simulink model "ICRA_demo_ver2"  (R2016a)
settings: Solver=FixedStepDiscrete  StartTime=0.0  StopTime=Inf  FixedStep=Ts  RelTol=1e-3
InitFcn:
  | Ts = 1/4000;
  | Ts2 = 1/1000;
  | Tmpc = 1/40;
  | 
  | q_off = calib.q_off;
  | q_init = calib.q_init;
libraries: xpcethercatlib x109, slrtlib x18
(part 2 of 2)

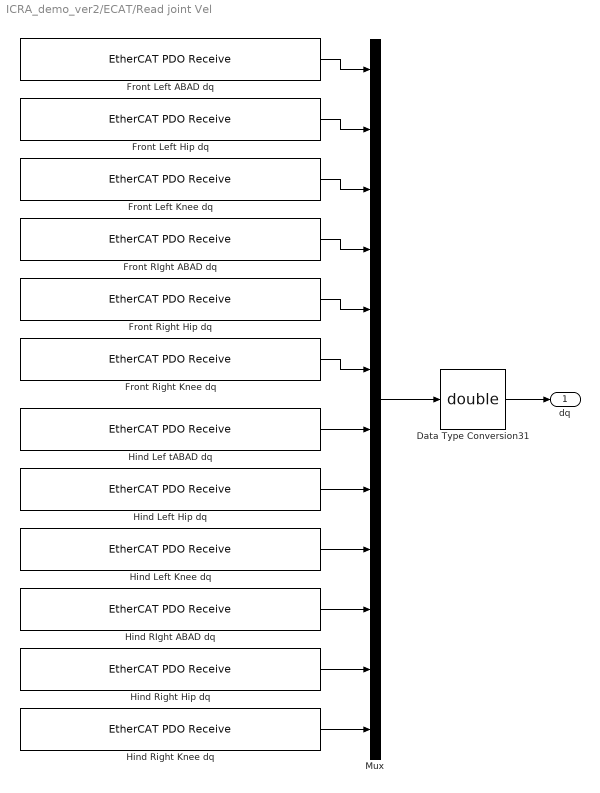
== system ICRA_demo_ver2/ECAT/Read joint Vel ==
  Data Type Conversion31 : DataTypeConversion  OutDataTypeStr=double
  Front Left ABAD dq : xpcethercatlib/EtherCAT PDO Receive  Priority=2  sig_name=Drive 1 (Elmo Drive).Inputs.Velocity actual value  sig_offset=920  sig_type=int32  type_size=32  sig_dim=1  device_id=0  sample_time=0.000250
  Front Left Hip dq : xpcethercatlib/EtherCAT PDO Receive  Priority=2  sig_name=Drive 2 (Elmo Drive).Inputs.Velocity actual value  sig_offset=1048  sig_type=int32  type_size=32  sig_dim=1  device_id=0  sample_time=0.000250
  Front Left Knee dq : xpcethercatlib/EtherCAT PDO Receive  Priority=2  sig_name=Drive 3 (Elmo Drive).Inputs.Velocity actual value  sig_offset=1176  sig_type=int32  type_size=32  sig_dim=1  device_id=0  sample_time=0.000250
  Front RIght ABAD dq : xpcethercatlib/EtherCAT PDO Receive  Priority=2  sig_name=Drive 13 (Elmo Drive).Inputs.Velocity actual value  sig_offset=2328  sig_type=int32  type_size=32  sig_dim=1  device_id=0  sample_time=0.000250
  Front Right Hip dq : xpcethercatlib/EtherCAT PDO Receive  Priority=2  sig_name=Drive 5 (Elmo Drive).Inputs.Velocity actual value  sig_offset=1304  sig_type=int32  type_size=32  sig_dim=1  device_id=0  sample_time=0.000250
  Front Right Knee dq : xpcethercatlib/EtherCAT PDO Receive  Priority=2  sig_name=Drive 6 (Elmo Drive).Inputs.Velocity actual value  sig_offset=1432  sig_type=int32  type_size=32  sig_dim=1  device_id=0  sample_time=0.000250
  Hind Lef tABAD dq : xpcethercatlib/EtherCAT PDO Receive  Priority=2  sig_name=Drive 7 (Elmo Drive).Inputs.Velocity actual value  sig_offset=1560  sig_type=int32  type_size=32  sig_dim=1  device_id=0  sample_time=0.000250
  Hind Left Hip dq : xpcethercatlib/EtherCAT PDO Receive  Priority=2  sig_name=Drive 8 (Elmo Drive).Inputs.Velocity actual value  sig_offset=1688  sig_type=int32  type_size=32  sig_dim=1  device_id=0  sample_time=0.000250
  Hind Left Knee dq : xpcethercatlib/EtherCAT PDO Receive  Priority=2  sig_name=Drive 9 (Elmo Drive).Inputs.Velocity actual value  sig_offset=1816  sig_type=int32  type_size=32  sig_dim=1  device_id=0  sample_time=0.000250
  Hind RIght ABAD dq : xpcethercatlib/EtherCAT PDO Receive  Priority=2  sig_name=Drive 10 (Elmo Drive).Inputs.Velocity actual value  sig_offset=1944  sig_type=int32  type_size=32  sig_dim=1  device_id=0  sample_time=0.000250
  Hind Right Hip dq : xpcethercatlib/EtherCAT PDO Receive  Priority=2  sig_name=Drive 11 (Elmo Drive).Inputs.Velocity actual value  sig_offset=2072  sig_type=int32  type_size=32  sig_dim=1  device_id=0  sample_time=0.000250
  Hind Right Knee dq : xpcethercatlib/EtherCAT PDO Receive  Priority=2  sig_name=Drive 12 (Elmo Drive).Inputs.Velocity actual value  sig_offset=2200  sig_type=int32  type_size=32  sig_dim=1  device_id=0  sample_time=0.000250
  Mux : Mux  Inputs=12
  dq : Outport
  wires:
  Hind Right Knee dq/1 -> Mux/12
  Hind Right Hip dq/1 -> Mux/11
  Hind RIght ABAD dq/1 -> Mux/10
  Hind Left Knee dq/1 -> Mux/9
  Hind Left Hip dq/1 -> Mux/8
  Hind Lef tABAD dq/1 -> Mux/7
  Front Right Knee dq/1 -> Mux/6
  Front Left Hip dq/1 -> Mux/2
  Front Left Knee dq/1 -> Mux/3
  Front RIght ABAD dq/1 -> Mux/4
  Front Right Hip dq/1 -> Mux/5
  Mux/1 -> Data Type Conversion31/1
  Data Type Conversion31/1 -> dq/1
  Front Left ABAD dq/1 -> Mux/1

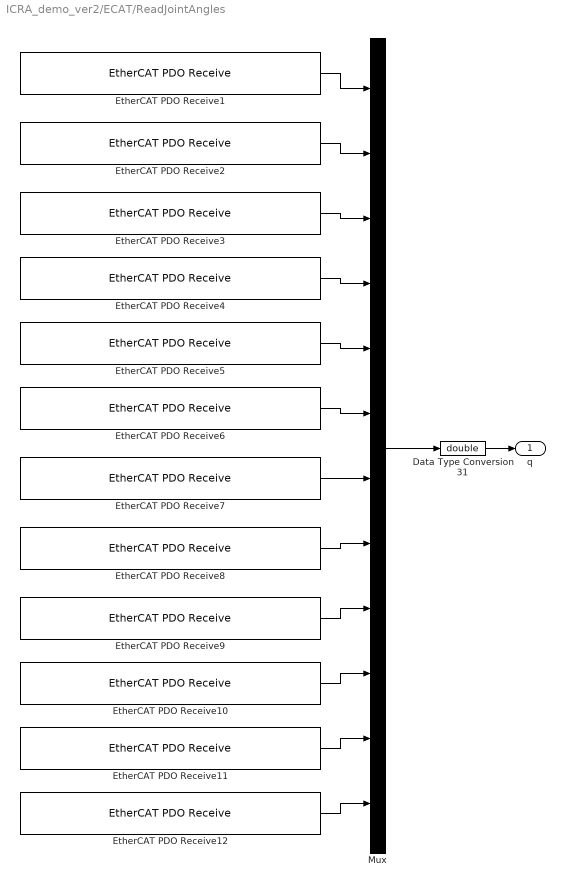
== system ICRA_demo_ver2/ECAT/ReadJointAngles ==
  Data Type Conversion31 : DataTypeConversion  OutDataTypeStr=double
  EtherCAT PDO Receive1 : xpcethercatlib/EtherCAT PDO Receive  Priority=2  sig_name=Drive 1 (Elmo Drive).Inputs.Position actual value  sig_offset=856  sig_type=int32  type_size=32  sig_dim=1  device_id=0  sample_time=0.000250
  EtherCAT PDO Receive10 : xpcethercatlib/EtherCAT PDO Receive  Priority=2  sig_name=Drive 10 (Elmo Drive).Inputs.Position actual value  sig_offset=1880  sig_type=int32  type_size=32  sig_dim=1  device_id=0  sample_time=0.000250
  EtherCAT PDO Receive11 : xpcethercatlib/EtherCAT PDO Receive  Priority=2  sig_name=Drive 11 (Elmo Drive).Inputs.Position actual value  sig_offset=2008  sig_type=int32  type_size=32  sig_dim=1  device_id=0  sample_time=0.000250
  EtherCAT PDO Receive12 : xpcethercatlib/EtherCAT PDO Receive  Priority=2  sig_name=Drive 12 (Elmo Drive).Inputs.Position actual value  sig_offset=2136  sig_type=int32  type_size=32  sig_dim=1  device_id=0  sample_time=0.000250
  EtherCAT PDO Receive2 : xpcethercatlib/EtherCAT PDO Receive  Priority=2  sig_name=Drive 2 (Elmo Drive).Inputs.Position actual value  sig_offset=984  sig_type=int32  type_size=32  sig_dim=1  device_id=0  sample_time=0.000250
  EtherCAT PDO Receive3 : xpcethercatlib/EtherCAT PDO Receive  Priority=2  sig_name=Drive 3 (Elmo Drive).Inputs.Position actual value  sig_offset=1112  sig_type=int32  type_size=32  sig_dim=1  device_id=0  sample_time=0.000250
  EtherCAT PDO Receive4 : xpcethercatlib/EtherCAT PDO Receive  Priority=2  sig_name=Drive 13 (Elmo Drive).Inputs.Position actual value  sig_offset=2264  sig_type=int32  type_size=32  sig_dim=1  device_id=0  sample_time=0.000250
  EtherCAT PDO Receive5 : xpcethercatlib/EtherCAT PDO Receive  Priority=2  sig_name=Drive 5 (Elmo Drive).Inputs.Position actual value  sig_offset=1240  sig_type=int32  type_size=32  sig_dim=1  device_id=0  sample_time=0.000250
  EtherCAT PDO Receive6 : xpcethercatlib/EtherCAT PDO Receive  Priority=2  sig_name=Drive 6 (Elmo Drive).Inputs.Position actual value  sig_offset=1368  sig_type=int32  type_size=32  sig_dim=1  device_id=0  sample_time=0.000250
  EtherCAT PDO Receive7 : xpcethercatlib/EtherCAT PDO Receive  Priority=2  sig_name=Drive 7 (Elmo Drive).Inputs.Position actual value  sig_offset=1496  sig_type=int32  type_size=32  sig_dim=1  device_id=0  sample_time=0.000250
  EtherCAT PDO Receive8 : xpcethercatlib/EtherCAT PDO Receive  Priority=2  sig_name=Drive 8 (Elmo Drive).Inputs.Position actual value  sig_offset=1624  sig_type=int32  type_size=32  sig_dim=1  device_id=0  sample_time=0.000250
  EtherCAT PDO Receive9 : xpcethercatlib/EtherCAT PDO Receive  Priority=2  sig_name=Drive 9 (Elmo Drive).Inputs.Position actual value  sig_offset=1752  sig_type=int32  type_size=32  sig_dim=1  device_id=0  sample_time=0.000250
  Mux : Mux  Inputs=12
  q : Outport
  wires:
  EtherCAT PDO Receive12/1 -> Mux/12
  EtherCAT PDO Receive11/1 -> Mux/11
  EtherCAT PDO Receive10/1 -> Mux/10
  EtherCAT PDO Receive9/1 -> Mux/9
  EtherCAT PDO Receive8/1 -> Mux/8
  EtherCAT PDO Receive7/1 -> Mux/7
  EtherCAT PDO Receive6/1 -> Mux/6
  EtherCAT PDO Receive1/1 -> Mux/1
  EtherCAT PDO Receive2/1 -> Mux/2
  EtherCAT PDO Receive3/1 -> Mux/3
  EtherCAT PDO Receive4/1 -> Mux/4
  EtherCAT PDO Receive5/1 -> Mux/5
  Mux/1 -> Data Type Conversion31/1
  Data Type Conversion31/1 -> q/1

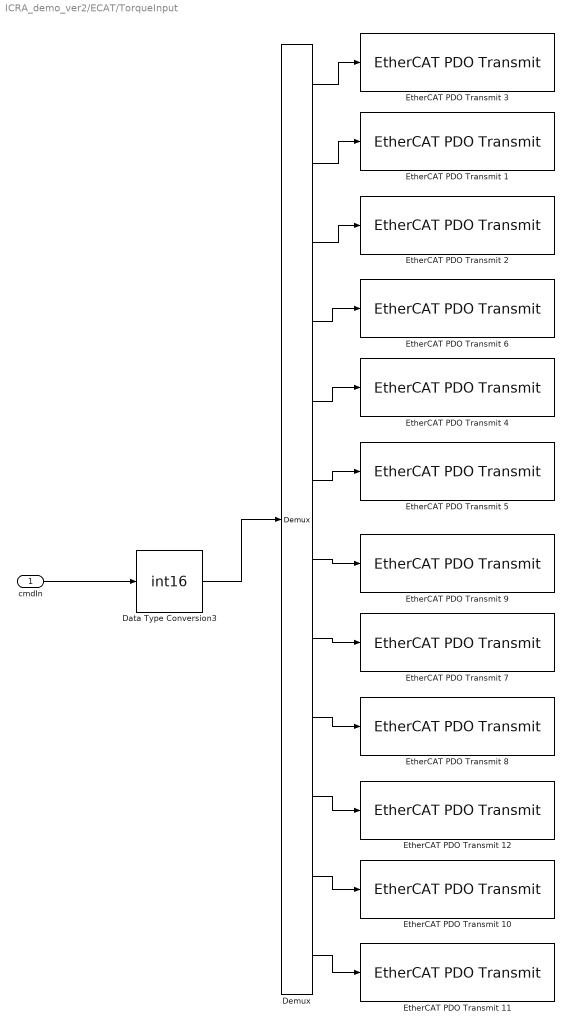
== system ICRA_demo_ver2/ECAT/TorqueInput ==
  cmdIn : Inport
  Data Type Conversion3 : DataTypeConversion  OutDataTypeStr=int16
  Demux : Demux  Outputs=12
  EtherCAT PDO Transmit 1 : xpcethercatlib/EtherCAT PDO Transmit   Priority=3  sig_name=Drive 2 (Elmo Drive).Outputs.Target Torque  sig_offset=1048  sig_type=int16  type_size=16  sig_dim=1  device_id=0  sample_time=0.000250
  EtherCAT PDO Transmit 10 : xpcethercatlib/EtherCAT PDO Transmit   Priority=3  sig_name=Drive 11 (Elmo Drive).Outputs.Target Torque  sig_offset=2072  sig_type=int16  type_size=16  sig_dim=1  device_id=0  sample_time=0.000250
  EtherCAT PDO Transmit 11 : xpcethercatlib/EtherCAT PDO Transmit   Priority=3  sig_name=Drive 12 (Elmo Drive).Outputs.Target Torque  sig_offset=2200  sig_type=int16  type_size=16  sig_dim=1  device_id=0  sample_time=0.000250
  EtherCAT PDO Transmit 12 : xpcethercatlib/EtherCAT PDO Transmit   Priority=3  sig_name=Drive 10 (Elmo Drive).Outputs.Target Torque  sig_offset=1944  sig_type=int16  type_size=16  sig_dim=1  device_id=0  sample_time=0.000250
  EtherCAT PDO Transmit 2 : xpcethercatlib/EtherCAT PDO Transmit   Priority=3  sig_name=Drive 3 (Elmo Drive).Outputs.Target Torque  sig_offset=1176  sig_type=int16  type_size=16  sig_dim=1  device_id=0  sample_time=0.000250
  EtherCAT PDO Transmit 3 : xpcethercatlib/EtherCAT PDO Transmit   Priority=3  sig_name=Drive 1 (Elmo Drive).Outputs.Target Torque  sig_offset=920  sig_type=int16  type_size=16  sig_dim=1  device_id=0  sample_time=0.000250
  EtherCAT PDO Transmit 4 : xpcethercatlib/EtherCAT PDO Transmit   Priority=3  sig_name=Drive 5 (Elmo Drive).Outputs.Target Torque  sig_offset=1304  sig_type=int16  type_size=16  sig_dim=1  device_id=0  sample_time=0.000250
  EtherCAT PDO Transmit 5 : xpcethercatlib/EtherCAT PDO Transmit   Priority=3  sig_name=Drive 6 (Elmo Drive).Outputs.Target Torque  sig_offset=1432  sig_type=int16  type_size=16  sig_dim=1  device_id=0  sample_time=0.000250
  EtherCAT PDO Transmit 6 : xpcethercatlib/EtherCAT PDO Transmit   Priority=3  sig_name=Drive 13 (Elmo Drive).Outputs.Target Torque  sig_offset=2328  sig_type=int16  type_size=16  sig_dim=1  device_id=0  sample_time=0.000250
  EtherCAT PDO Transmit 7 : xpcethercatlib/EtherCAT PDO Transmit   Priority=3  sig_name=Drive 8 (Elmo Drive).Outputs.Target Torque  sig_offset=1688  sig_type=int16  type_size=16  sig_dim=1  device_id=0  sample_time=0.000250
  EtherCAT PDO Transmit 8 : xpcethercatlib/EtherCAT PDO Transmit   Priority=3  sig_name=Drive 9 (Elmo Drive).Outputs.Target Torque  sig_offset=1816  sig_type=int16  type_size=16  sig_dim=1  device_id=0  sample_time=0.000250
  EtherCAT PDO Transmit 9 : xpcethercatlib/EtherCAT PDO Transmit   Priority=3  sig_name=Drive 7 (Elmo Drive).Outputs.Target Torque  sig_offset=1560  sig_type=int16  type_size=16  sig_dim=1  device_id=0  sample_time=0.000250
  wires:
  Demux/3 -> EtherCAT PDO Transmit 2/1
  Demux/2 -> EtherCAT PDO Transmit 1/1
  Demux/1 -> EtherCAT PDO Transmit 3/1
  cmdIn/1 -> Data Type Conversion3/1
  Data Type Conversion3/1 -> Demux/1
  Demux/4 -> EtherCAT PDO Transmit 6/1
  Demux/5 -> EtherCAT PDO Transmit 4/1
  Demux/6 -> EtherCAT PDO Transmit 5/1
  Demux/7 -> EtherCAT PDO Transmit 9/1
  Demux/8 -> EtherCAT PDO Transmit 7/1
  Demux/9 -> EtherCAT PDO Transmit 8/1
  Demux/10 -> EtherCAT PDO Transmit 12/1
  Demux/11 -> EtherCAT PDO Transmit 10/1
  Demux/12 -> EtherCAT PDO Transmit 11/1

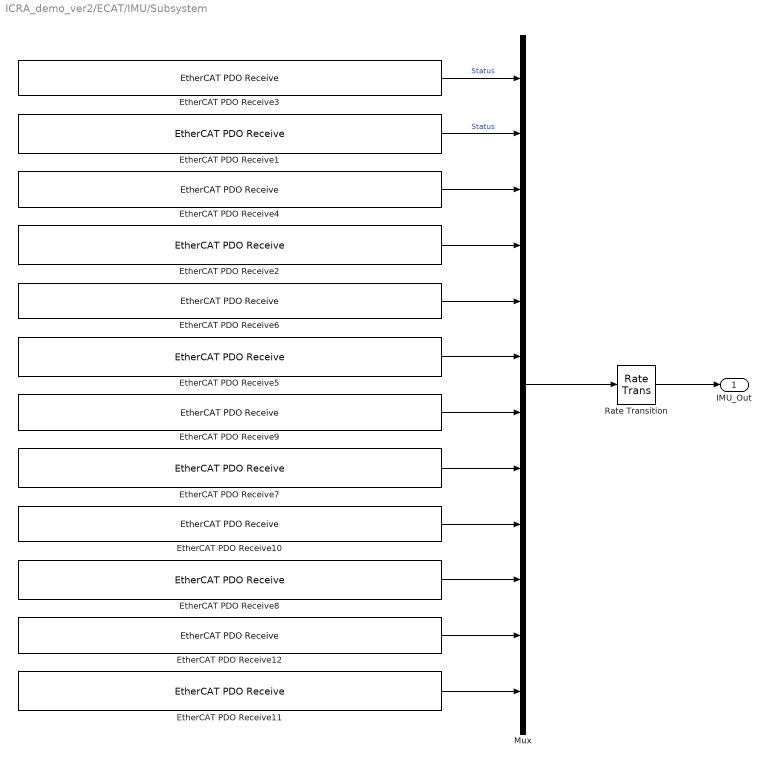
== system ICRA_demo_ver2/ECAT/IMU/Subsystem ==
  EtherCAT PDO Receive1 : xpcethercatlib/EtherCAT PDO Receive  Priority=2  sig_name=Box 4 (XMC4800 Generic Ethercat Slave).IN_GENERIC process data mapping.IN_GEN_INT2  sig_offset=584  sig_type=uint16  type_size=16  sig_dim=1  device_id=0  sample_time=0.000250
  EtherCAT PDO Receive10 : xpcethercatlib/EtherCAT PDO Receive  Priority=2  sig_name=Box 4 (XMC4800 Generic Ethercat Slave).IN_GENERIC process data mapping.IN_GEN_Bit5  sig_offset=696  sig_type=uint16  type_size=16  sig_dim=1  device_id=0  sample_time=0.000250
  EtherCAT PDO Receive11 : xpcethercatlib/EtherCAT PDO Receive  Priority=2  sig_name=Box 4 (XMC4800 Generic Ethercat Slave).IN_GENERIC process data mapping.IN_GEN_Bit8  sig_offset=744  sig_type=uint16  type_size=16  sig_dim=1  device_id=0  sample_time=0.000250
  EtherCAT PDO Receive12 : xpcethercatlib/EtherCAT PDO Receive  Priority=2  sig_name=Box 4 (XMC4800 Generic Ethercat Slave).IN_GENERIC process data mapping.IN_GEN_Bit7  sig_offset=728  sig_type=uint16  type_size=16  sig_dim=1  device_id=0  sample_time=0.000250
  EtherCAT PDO Receive2 : xpcethercatlib/EtherCAT PDO Receive  Priority=2  sig_name=Box 4 (XMC4800 Generic Ethercat Slave).IN_GENERIC process data mapping.IN_GEN_INT4  sig_offset=616  sig_type=uint16  type_size=16  sig_dim=1  device_id=0  sample_time=0.000250
  EtherCAT PDO Receive3 : xpcethercatlib/EtherCAT PDO Receive  Priority=2  sig_name=Box 4 (XMC4800 Generic Ethercat Slave).IN_GENERIC process data mapping.IN_GEN_INT1  sig_offset=568  sig_type=uint16  type_size=16  sig_dim=1  device_id=0  sample_time=0.000250
  EtherCAT PDO Receive4 : xpcethercatlib/EtherCAT PDO Receive  Priority=2  sig_name=Box 4 (XMC4800 Generic Ethercat Slave).IN_GENERIC process data mapping.IN_GEN_INT3  sig_offset=600  sig_type=uint16  type_size=16  sig_dim=1  device_id=0  sample_time=0.000250
  EtherCAT PDO Receive5 : xpcethercatlib/EtherCAT PDO Receive  Priority=2  sig_name=Box 4 (XMC4800 Generic Ethercat Slave).IN_GENERIC process data mapping.IN_GEN_Bit2  sig_offset=648  sig_type=uint16  type_size=16  sig_dim=1  device_id=0  sample_time=0.000250
  EtherCAT PDO Receive6 : xpcethercatlib/EtherCAT PDO Receive  Priority=2  sig_name=Box 4 (XMC4800 Generic Ethercat Slave).IN_GENERIC process data mapping.IN_GEN_Bit1  sig_offset=632  sig_type=uint16  type_size=16  sig_dim=1  device_id=0  sample_time=0.000250
  EtherCAT PDO Receive7 : xpcethercatlib/EtherCAT PDO Receive  Priority=2  sig_name=Box 4 (XMC4800 Generic Ethercat Slave).IN_GENERIC process data mapping.IN_GEN_Bit4  sig_offset=680  sig_type=uint16  type_size=16  sig_dim=1  device_id=0  sample_time=0.000250
  EtherCAT PDO Receive8 : xpcethercatlib/EtherCAT PDO Receive  Priority=2  sig_name=Box 4 (XMC4800 Generic Ethercat Slave).IN_GENERIC process data mapping.IN_GEN_Bit6  sig_offset=712  sig_type=uint16  type_size=16  sig_dim=1  device_id=0  sample_time=0.000250
  EtherCAT PDO Receive9 : xpcethercatlib/EtherCAT PDO Receive  Priority=2  sig_name=Box 4 (XMC4800 Generic Ethercat Slave).IN_GENERIC process data mapping.IN_GEN_Bit3  sig_offset=664  sig_type=uint16  type_size=16  sig_dim=1  device_id=0  sample_time=0.000250
  Mux : Mux  Inputs=12
  Rate Transition : RateTransition  Deterministic=off  OutPortSampleTime=Ts2
  IMU_Out : Outport
  wires:
  EtherCAT PDO Receive1/1 -> Mux/2  "Status"
  EtherCAT PDO Receive7/1 -> Mux/8
  EtherCAT PDO Receive12/1 -> Mux/11
  EtherCAT PDO Receive11/1 -> Mux/12
  Mux/1 -> Rate Transition/1
  EtherCAT PDO Receive3/1 -> Mux/1  "Status"
  EtherCAT PDO Receive4/1 -> Mux/3
  EtherCAT PDO Receive6/1 -> Mux/5
  EtherCAT PDO Receive8/1 -> Mux/10
  EtherCAT PDO Receive9/1 -> Mux/7
  EtherCAT PDO Receive5/1 -> Mux/6
  EtherCAT PDO Receive10/1 -> Mux/9
  EtherCAT PDO Receive2/1 -> Mux/4
  Rate Transition/1 -> IMU_Out/1

== matlab function ICRA_demo_ver2/ECAT/IMU/MATLAB Function ==
  data: IMU_Out input; AccelX output; AccelY output; AccelZ output; GyroX output; GyroY output; GyroZ output
function [AccelX, AccelY, AccelZ, GyroX, GyroY, GyroZ] = fcn(IMU_Out)

AccelX_Low = dec2bin( IMU_Out(1), 16 );
AccelX_High = dec2bin( IMU_Out(2), 16 );
AccelY_Low = dec2bin( IMU_Out(3), 16 );
AccelY_High = dec2bin( IMU_Out(4), 16 );
AccelZ_Low = dec2bin( IMU_Out(5), 16 );
AccelZ_High = dec2bin( IMU_Out(6), 16 );
GyroX_Low = dec2bin( IMU_Out(7), 16 );
GyroX_High = dec2bin( IMU_Out(8), 16 );
GyroY_Low = dec2bin( IMU_Out(9), 16 );
GyroY_High = dec2bin( IMU_Out(10), 16 );
GyroZ_Low = dec2bin( IMU_Out(11), 16 );
GyroZ_High = dec2bin( IMU_Out(12), 16 );

AccelX_bin = [ AccelX_High, AccelX_Low ];
AccelY_bin = [ AccelY_High, AccelY_Low ];
AccelZ_bin = [ AccelZ_High, AccelZ_Low ];
GyroX_bin = [ GyroX_High, GyroX_Low ];
GyroY_bin = [ GyroY_High, GyroY_Low ];
GyroZ_bin = [ GyroZ_High, GyroZ_Low ];

AccelX= typecast( uint32( bin2dec( AccelX_bin ) ), 'single' );
AccelY= typecast( uint32( bin2dec( AccelY_bin ) ), 'single' );
AccelZ= typecast( uint32( bin2dec( AccelZ_bin ) ), 'single' );
GyroX= typecast( uint32( bin2dec( GyroX_bin ) ), 'single' );
GyroY= typecast( uint32( bin2dec( GyroY_bin ) ), 'single' );
GyroZ= typecast( uint32( bin2dec( GyroZ_bin ) ), 'single' );

== matlab function ICRA_demo_ver2/ECAT/IMU/MATLAB Function1 ==
  data: vin input; vout output; vR_change input
function vout = fcn(vin,vR_change)

R_change = reshape(vR_change,[3,3]);

vout = R_change * vin;

end

== matlab function ICRA_demo_ver2/MATLAB Function ==
  data: vRyaw input; J_f_b input; u input; tau output; dq_all input; a_all input; flag_tau input; flag_f_comp input; c_50 input; c_25 input
function tau = ...
    fcn(vRyaw,J_f_b,u,dq_all,a_all,flag_tau,flag_f_comp,c_50,c_25)

% motor constants
K50 = c_50 * 190;
K25 = c_25 * 350;

Ryaw = reshape(vRyaw,[3,3]);

tau = zeros(12,1);

for i_leg = 1:4
    idx = 3*(i_leg-1) + (1:3);
    F = - u (idx);
    J = reshape(J_f_b(9*(i_leg-1) + (1:9)),[3,3]);
    tau(idx) = J' * (Ryaw' * F);
    
    % friction compensation
    tau_f_comp = a_all(idx) .* dq_all(idx);
    tau(idx) = flag_tau * tau(idx) + flag_f_comp * tau_f_comp;

end

% ABAD
tau([1,4,7,10]) = K25 * tau([1,4,7,10]);

idx_ = [2,3,5,6,8,9,11,12];
tau(idx_) = K50 * tau(idx_);


end

== matlab function ICRA_demo_ver2/MATLAB Function1 ==
  data: t input; xop input; vop input; vR input; vRyaw input; wop input; fop input; r_COM_yaw_i input; Q_co input; Qf_co input; R_co input; p_ref input; npr output; mpr output; ppr output; lpr output; nconespr output; qintpr output; nexcpr output; G output; cpr output; hpr output; ex output; ev output; eR output; ew output; vJ input; mass input; vpf output; xd output
function [npr,mpr,ppr,lpr,nconespr,qintpr,nexcpr,G,cpr,hpr,...
          ex,ev,eR,ew,vpf,xd] = ...
    formulate(t,xop,vop,vR,vRyaw,wop,fop,r_COM_yaw_i,Q_co,Qf_co,R_co,p_ref,vJ,mass)

%%% error = F_L*(d_u) + F_C;
%%% F_L := proportional term
%%% F_C := constant term

dt = 1/40;
Ryaw = reshape(vRyaw,[3,3]);
R = reshape(vR,[3,3]);
J = diag(vJ);
Horizon = 7;
g = 9.81;
mu = 1;

% reference trajectory
enable_x = p_ref(1);
enable_z = p_ref(2);
enable_th = p_ref(3);
f_x = p_ref(4);
f_z = p_ref(5);
f_th = p_ref(6);
A_x = p_ref(7);
A_z = p_ref(8);
A_th = p_ref(9);
bias_z = p_ref(10);

% desired state
x_d = enable_x * A_x * sin(f_x * t);
z_d = enable_z * A_z * sin(f_z * t) + bias_z;
th_d = enable_th * A_th * sin(f_th * t);

dx_d = A_x * f_x * cos(f_x * t);
dz_d = A_z * f_z * cos(f_z * t);
dth_d = A_th * f_th * cos(f_th * t);


%% 
if t < 10
    Ryaw = reshape(eye(3),[],1);
    wop = [0;0;0];
    vop = [0;0;0];
    fop = [0;0;mass*g/4;0;0;mass*g/4;0;0;mass*g/4;0;0;mass*g/4];
    xop = [0;0;0.15];
    vpf = [0.15;0.08;0;0.15;-0.08;0;-0.15;0.08;0;-0.15;-0.08;0];
else
    vpf = [xop;xop;xop;xop] - r_COM_yaw_i;
end

%% desired state
% theta: pitch angle
Rd = [cos(th_d),0,sin(th_d);...
      0,1,0;...
      -sin(th_d),0,cos(th_d)];
% Rd = eye(3);
  
wd = [0;dth_d;0];
xd = [x_d;0;z_d];
vd = [dx_d;0;dz_d];
pf = reshape(vpf,[3,4]);

%% error
ex = xop - xd;
ev = vop - vd;
% eR = 1/2 * veeMap(Rd' * Ryaw - Ryaw' * Rd);
eR = 1/2 * veeMap(Rd' * R - R' * Rd);
ew = wop - Ryaw' * Rd * wd;


%%% Error Gains
Q = diag([repmat(Q_co,[Horizon-1,1]);Qf_co]);
% Qf = diag(Qf_co);
% Q(end-Horizon+1:end,end-Horizon+1:end) = Qf;

%%% Control Gains
% R_co = 0.1*ones(12,1);
R = diag(repmat(R_co,[Horizon,1]));

%%% Desired/Reference Control Input
Ud = [0;0;mass*g/4;0;0;mass*g/4;0;0;mass*g/4;0;0;mass*g/4];
Constant = repmat(fop-Ud,[Horizon,1]);


[A,B,D]=complete(dt,Ryaw,wop,fop,xop,pf,J,mass,g);


q0 = [xop;vop;Ryaw(:);wop];

P = [1,0,0,0,0,0,0,0,0;0,0,0,1,0,0,0,0,0;0,0,0,0,0,0,1,0,0;0,1,0,0,0,0,0,0,0;0,0,0,0,1,0,0,0,0;0,0,0,0,0,0,0,1,0;0,0,1,0,0,0,0,0,0;0,0,0,0,0,1,0,0,0;0,0,0,0,0,0,0,0,1];
L = 0.5*(kron(eye(3),Rd')-(kron(Rd',eye(3))*P));

Vmap = [0 0 0 0 0 1 0 0 0;0 0 -1 0 0 0 0 0 0;0 1 0 0 0 0 0 0 0];
F_Rdwd = calculate_F(Rd*wd);

TT12 = [eye(6),zeros(6,12)];
TT3 = [zeros(9,6),eye(9),zeros(9,3)];
TT4 = [zeros(3,15),eye(3)];

X = [TT12;Vmap*L*TT3;TT4 - F_Rdwd*TT3];
F_C = zeros(12*Horizon,1);
L = (A*q0)+D;

for i = 1:Horizon
    idx = [1:12]+12*(i-1);
    idy = 1:(12*i);
    
%     F_L(idx,idy) = X*[A*F_L(1:idx-12,idy-12),B];
    F_C(idx,1) = X*L;
    
    L = A*L + D;
   
end

F_L = [X*B,zeros(12,12*6);...
       X*A*B,X*B,zeros(12,12*5);...
       X*A^2*B,X*A*B,X*B,zeros(12,12*4);...
       X*A^3*B,X*A^2*B,X*A*B,X*B,zeros(12,12*3);...
       X*A^4*B,X*A^3*B,X*A^2*B,X*A*B,X*B,zeros(12,12*2);...
       X*A^5*B,X*A^4*B,X*A^3*B,X*A^2*B,X*A*B,X*B,zeros(12,12*1);...
       X*A^6*B,X*A^5*B,X*A^4*B,X*A^3*B,X*A^2*B,X*A*B,X*B];



F_C = F_C - repmat([xd;vd;zeros(6,1)],[Horizon,1]);



H = 2*((F_L'*Q*F_L) + R);
f = 2*(F_C'*Q*F_L + Constant'*R);


W = chol(H,'upper');

ncones = 1;

G1 = [f./sqrt(2),-1/sqrt(2);...
        -W,zeros(size(H,1),1);...
      -f./sqrt(2),1/sqrt(2)];
  
h1 = 1/sqrt(2)*[1;zeros(size(H,1),1);1];

G_int = zeros(12*Horizon,(12*Horizon)+1);
C = [0 0 mu];
A = [1 0 0;0 1 0];

for i = 1:Horizon
    for ct = 1:4
        ncones = ncones + 1;
        idx = [1:3] + 3*(ct-1) + 12*(i-1);
        idy = [1:3] + 3*(ct-1) + 12*(i-1);
        G_int(idx,idy) = [-C;-A];
    end
end

G_h = [mu*fop(3);fop(1:2);mu*fop(6);fop(4:5);mu*fop(9);fop(7:8);mu*fop(12);fop(10:11)];
hpr = [h1;repmat(G_h,[Horizon,1])];

G1 = [G1;G_int];
G=G1(:);

npr = (12*Horizon)+1;
mpr = size(G,1)/npr;
ppr = 0;
lpr = 0;
nconespr = ncones;
qintpr = zeros(Horizon*12 + 1,1);
qintpr(1) = size(W,1) + 2;qintpr(2:ncones) = 3*ones(4*Horizon,1);
nexcpr = 0;
cpr = [zeros(12*Horizon,1);1];

end

function s = veeMap(S)
    s = zeros(3,1);
    s(2,1) = S(1,3);
    s(1,1) = S(3,2);
    s(3,1) = S(2,1);
end

== matlab function ICRA_demo_ver2/safety1 ==
  data: sat input; tau_calc input; y output
function y = fcn(sat,tau_calc)

sat_ = zeros(12,1);
sat_(1:3) = sat(1);
sat_(4:6) = sat(2);
sat_(7:9) = sat(3);
sat_(10:12) = sat(4);


% leg saturation
y = tau_calc;
y(tau_calc >= sat_) = sat_(tau_calc >= sat_);
y(tau_calc <= -sat_) = -sat_(tau_calc <= -sat_);


end

== matlab function ICRA_demo_ver2/ECAT/MATLAB Function4 ==
  data: vin input; vout output; direction input; Permu input
function vout = fcn(vin,direction,Permu)

k = 1/8192*2*pi/23.3594;        % count to [rad]

vout = k * vin .* direction;

vout = Permu * vout;

end

== matlab function ICRA_demo_ver2/ECAT/Ratio ==
  data: tau_real_cmd input; tau_out output
function tau_out  = Cmd2Torque(tau_real_cmd)
% ---  define ratios between output torque and current cmd ---
k4450_pos = 0.0048891;
k4450_neg = 0.0047417;
% k4425_pos = 0.0025844;
% k4425_neg = 0.0025505;

tau_real_cmd(tau_real_cmd<0) = tau_real_cmd(tau_real_cmd<0)*k4450_neg;
tau_real_cmd(tau_real_cmd>0) = tau_real_cmd(tau_real_cmd>0)*k4450_pos;

tau_out = tau_real_cmd;

end

== matlab function ICRA_demo_ver2/ECAT/Enable Elmo/State switch2 ==
  data: time input; ctrl output uint16; MaxTau output uint16; enable input; mode output int8
function [ctrl,MaxTau,mode] = fcn(time, enable)
% This is stupid!!! Seems like EtherCAT won't be ready in the first 2s
% after simulation starts... This thing took me 3 hours!!!
% Chad, 2016.08.12

persistent phase t_switch

if isempty(phase)
    phase = 1;
    t_switch = 9527;
end

if time>0.1
    t_switch(enable==1) = time;
end

if phase==1 && time-t_switch>0.1
    phase = phase + 1;
elseif phase==2 && time-t_switch>0.15
    phase = phase + 1;
elseif phase==3 && enable==1
    phase = phase + 1;
elseif phase==4 && enable==1
    phase = phase - 1;
end

mode = int8(10);

if phase==1
    % Fault Reset
    ctrl = uint16(128);
    MaxTau = uint16(0);
elseif phase==2
    % Trans 2
    ctrl = uint16(6);
    MaxTau = uint16(0);
elseif phase==3
    % Trans 3+4
    ctrl = uint16(15);
    MaxTau = uint16(2000);
elseif phase==4
    % Trans 5
    ctrl = uint16(7);
    MaxTau = uint16(0);
else
    ctrl = uint16(128);
    MaxTau = uint16(0);
end

== matlab function ICRA_demo_ver2/ECAT/IMU/MATLAB Function2 ==
  data: t input size=1; Accelerometer input; Gyroscope input; q_IMU output size=3; Quat_IMU output size=4; vR output size=9; e_dir output size=3; Kp input size=1; vR_yaw output; Drift input
% function [q_IMU,dyaw,e_dir,Quat_IMU] = fcn(Accelerometer,Gyroscope)
function [ q_IMU, Quat_IMU, vR,e_dir,vR_yaw ] = ...
    fcn( t, Accelerometer, Gyroscope, Kp,Drift)
%#codegen
persistent Quaternion eInt Quaternion_yaw
if isempty(Quaternion)
    Quaternion = [1 0 0 0];
    Quaternion_yaw = [1 0 0 0];
%    Quaternion = [sqrt(2)/2         0         0    sqrt(2)/2];
    eInt = zeros(3,1);
end
Ki = 0.0;
SamplePeriod = 1/1000;

q = Quaternion;
q_yaw = Quaternion_yaw;
% Normalise accelerometer measurement
Accelerometer = Accelerometer / my_norm(Accelerometer);	% normalise magnitude

% Estimated direction of gravity and magnetic flux
v = [2*(q(2)*q(4) - q(1)*q(3)),
    2*(q(1)*q(2) + q(3)*q(4)),
    q(1)^2 - q(2)^2 - q(3)^2 + q(4)^2];

% Error is sum of cross product between estimated direction and measured direction of field
if t <5
    % Error somehow started with NaN. This prevents that from happening
    e_dir = zeros(3,1);
else
    e_dir = my_cross(Accelerometer, v);
end
eInt = eInt + e_dir * SamplePeriod;

% Apply feedback terms
dyaw = Gyroscope(3);
Gyroscope = Gyroscope + Kp * e_dir + Ki * eInt;
% Compute rate of change of quaternion
qDot = 0.5 * quaternProd(q, [0 Gyroscope(1) Gyroscope(2) Gyroscope(3)]);
qDot(4) = qDot(4)+Drift;
% Integrate to yield quaternion
q = q + qDot * SamplePeriod;
q_yaw = q_yaw + [1 1 1 0].*qDot * SamplePeriod;

Quaternion = q / my_norm_quat(q); % normalise quaternion\
Quaternion_yaw = q_yaw / my_norm_quat(q_yaw); % normalise quaternion\
[q_IMU]= quatToRpy((Quaternion));
Quat_IMU = zeros(4,1);
R = zeros(3,3);
R(1,1) = Quaternion(1)^2+Quaternion(2)^2-Quaternion(3)^2-Quaternion(4)^2;
R(1,2) = 2*(Quaternion(2)*Quaternion(3)-Quaternion(1)*Quaternion(4));
R(1,3) = 2*(Quaternion(1)*Quaternion(3)+Quaternion(2)*Quaternion(4));
R(2,2) = Quaternion(1)^2-Quaternion(2)^2+Quaternion(3)^2-Quaternion(4)^2;
R(2,3) = 2*(Quaternion(3)*Quaternion(4)-Quaternion(1)*Quaternion(2));
R(3,3) = Quaternion(1)^2-Quaternion(2)^2-Quaternion(3)^2+Quaternion(4)^2;
R(2,1) = 2*(Quaternion(1)*Quaternion(4)+Quaternion(2)*Quaternion(3));
R(3,1) = 2*(Quaternion(2)*Quaternion(4)-Quaternion(1)*Quaternion(3));
R(3,2) = 2*(Quaternion(1)*Quaternion(2)+Quaternion(3)*Quaternion(4));

R_yaw = zeros(3,3);
R_yaw(1,1) = Quaternion_yaw(1)^2+Quaternion_yaw(2)^2-Quaternion_yaw(3)^2-Quaternion_yaw(4)^2;
R_yaw(1,2) = 2*(Quaternion_yaw(2)*Quaternion_yaw(3)-Quaternion_yaw(1)*Quaternion_yaw(4));
R_yaw(1,3) = 2*(Quaternion_yaw(1)*Quaternion_yaw(3)+Quaternion_yaw(2)*Quaternion_yaw(4));
R_yaw(2,2) = Quaternion_yaw(1)^2-Quaternion_yaw(2)^2+Quaternion_yaw(3)^2-Quaternion_yaw(4)^2;
R_yaw(2,3) = 2*(Quaternion_yaw(3)*Quaternion_yaw(4)-Quaternion_yaw(1)*Quaternion_yaw(2));
R_yaw(3,3) = Quaternion_yaw(1)^2-Quaternion_yaw(2)^2-Quaternion_yaw(3)^2+Quaternion_yaw(4)^2;
R_yaw(2,1) = 2*(Quaternion_yaw(1)*Quaternion_yaw(4)+Quaternion_yaw(2)*Quaternion_yaw(3));
R_yaw(3,1) = 2*(Quaternion_yaw(2)*Quaternion_yaw(4)-Quaternion_yaw(1)*Quaternion_yaw(3));
R_yaw(3,2) = 2*(Quaternion_yaw(1)*Quaternion_yaw(2)+Quaternion_yaw(3)*Quaternion_yaw(4));

vR = reshape(R,[9,1]);
vR_yaw = reshape(R_yaw,[9,1]);

Quat_IMU(1) = Quaternion(1);
Quat_IMU(2) = Quaternion(2);
Quat_IMU(3) = Quaternion(3);
Quat_IMU(4) = Quaternion(4);

== matlab function ICRA_demo_ver2/ECAT/IMU/MATLAB Function3 ==
  data: vin input; vout output; vR_change input
function vout = fcn(vin,vR_change)

R_change = reshape(vR_change,[3,3]);

vout = R_change * vin;

end

== matlab function ICRA_demo_ver2/ECAT/MATLAB Function1 ==
  data: q_raw input; q_off input; q_init input; q output; direction input; Permu input
function q = fcn(q_raw,q_off,q_init,direction,Permu)

% count to [rad]
k = 1/8192*2*pi/23.3594;        

temp = (Permu * (q_raw - q_off)) .* direction;

% [count] to [rad]
q = k * temp + q_init / 180 * pi;


end

== matlab function ICRA_demo_ver2/ECAT/MATLAB Function3 ==
  data: vin input; vout output; direction input; Permu input
function vout = fcn(vin,direction,Permu)

k = 1/8192*2*pi/23.3594;        % count to [rad]

vout = k * vin .* direction;

vout = Permu * vout;

end

== matlab function ICRA_demo_ver2/MATLAB Function2 ==
  data: t input; y output; u input
function y = fcn(t,u)
%#codegen
if t<=10
    y = zeros(12,1);    
else
    y = u;
end

== matlab function ICRA_demo_ver2/MATLAB Function3 ==
  data: u input; y output; r input
function y = fcn(u,r)


y = Vec_to_Skew(-r(1:3))*u(1:3)+Vec_to_Skew(-r(4:6))*u(4:6)+Vec_to_Skew(-r(7:9))*u(7:9)+Vec_to_Skew(-r(10:12))*u(10:12);
% M = zeros
% for i_leg = 1:4
%     idx = (1:3) + (i_leg-1)*3;
%     rr = r(idx);
%     uu  = u(idx);
%     
%     
%     
%     
%     
%     
%     
%     
%     
%     
% end

== matlab function ICRA_demo_ver2/ECAT/MATLAB Function5 ==
  data: vin input; vout output; direction input
function vout = fcn(vin,direction)

invP = ...
    [0     0     0     0     0     0     0     0     0     0     1     0;
     0     0     0     0     0     0     0     0     0     0     0     1;
     0     0     0     0     0     0     0     0     0     1     0     0;
     0     1     0     0     0     0     0     0     0     0     0     0;
     0     0     0     1     0     0     0     0     0     0     0     0;
     0     0     0     0     0     1     0     0     0     0     0     0;
     0     0     0     0     1     0     0     0     0     0     0     0;
     0     0     0     0     0     0     0     1     0     0     0     0;
     0     0     0     0     0     0     0     0     1     0     0     0;
     0     0     0     0     0     0     1     0     0     0     0     0;
     1     0     0     0     0     0     0     0     0     0     0     0;
     0     0     1     0     0     0     0     0     0     0     0     0];


temp = vin .* direction;
vout = invP * temp;

end

== matlab function ICRA_demo_ver2/ECAT/permutate3 ==
  data: vin input; vout output; Permu input
function vout = fcn(vin,Permu)

vout = Permu * vin;

end

== matlab function ICRA_demo_ver2/ECAT/IMU/Estimate X ==
  data: t input; p_COM_est output; velCOM_filt input; Kp_x input; phase input; r_COM_yaw_avg input; r_COM_yaw_i input; p1_out output; p2_out output; p3_out output; p4_out output
function [p_COM_est,p1_out,p2_out,p3_out,p4_out] = ...
    fcn_est_x(t,velCOM_filt,Kp_x,phase,r_COM_yaw_avg,r_COM_yaw_i)

Ts2 = 1/1000;

r_COM_yaw_1 = r_COM_yaw_i(1:3);
r_COM_yaw_2 = r_COM_yaw_i(4:6);
r_COM_yaw_3 = r_COM_yaw_i(7:9);
r_COM_yaw_4 = r_COM_yaw_i(10:12);

persistent x_est p1_est p2_est p3_est p4_est
if isempty(x_est)
    x_est = [0;0;0];
    p1_est = r_COM_yaw_avg - r_COM_yaw_1;
    p2_est = r_COM_yaw_avg - r_COM_yaw_2;
    p3_est = r_COM_yaw_avg - r_COM_yaw_3;
    p4_est = r_COM_yaw_avg - r_COM_yaw_4;
end

if (t < 5)
    p1_est = r_COM_yaw_avg - r_COM_yaw_1;
    p2_est = r_COM_yaw_avg - r_COM_yaw_2;
    p3_est = r_COM_yaw_avg - r_COM_yaw_3;
    p4_est = r_COM_yaw_avg - r_COM_yaw_4;
end


%% x estimation

if (t < 5)
    e_x = zeros(3,1);
    e_x1 = zeros(3,1);
    e_x2 = zeros(3,1);
    e_x3 = zeros(3,1);
    e_x4 = zeros(3,1);
    xdot = zeros(3,1);
else
    if phase == 1
        e_x = (x_est - p1_est) - r_COM_yaw_1;
        xdot = velCOM_filt - Kp_x * e_x;
    elseif phase == 2
        e_x = (x_est - p2_est) - r_COM_yaw_2;
        xdot = velCOM_filt - Kp_x * e_x;
    elseif phase == 3
        e_x = (x_est - p3_est) - r_COM_yaw_3;
        xdot = velCOM_filt - Kp_x * e_x;
    elseif phase == 4
        e_x = (x_est - p4_est) - r_COM_yaw_4;
        xdot = velCOM_filt - Kp_x * e_x;
    elseif phase == 6
        e_x1 = (x_est - p1_est) - r_COM_yaw_1;
        e_x2 = (x_est - p2_est) - r_COM_yaw_2;
        e_x3 = (x_est - p3_est) - r_COM_yaw_3;
        e_x4 = (x_est - p4_est) - r_COM_yaw_4;
        xdot = velCOM_filt - 1/4 * Kp_x * (e_x1 + e_x2 + e_x3 + e_x4);
    else
        xdot = velCOM_filt;
    end
end

x_est = x_est + xdot * Ts2;

p_COM_est = x_est;
p1_out = p1_est;
p2_out = p2_est;
p3_out = p3_est;
p4_out = p4_est;

end

== matlab function ICRA_demo_ver2/ECAT/MATLAB Function ==
  data: P output
function P = fcn()
P = ...
    [0     0     0     0     0     0     0     0     0     0     1     0;
     0     0     0     1     0     0     0     0     0     0     0     0;
     0     0     0     0     0     0     0     0     0     0     0     1;
     0     0     0     0     1     0     0     0     0     0     0     0;
     0     0     0     0     0     0     1     0     0     0     0     0;
     0     0     0     0     0     1     0     0     0     0     0     0;
     0     0     0     0     0     0     0     0     0     1     0     0;
     0     0     0     0     0     0     0     1     0     0     0     0;
     0     0     0     0     0     0     0     0     1     0     0     0;
     0     0     1     0     0     0     0     0     0     0     0     0;
     1     0     0     0     0     0     0     0     0     0     0     0;
     0     1     0     0     0     0     0     0     0     0     0     0];

== matlab function ICRA_demo_ver2/ECAT/IMU/EstimateVelFromIMU ==
  data: t input; vel_COM_yaw_avg input; vel_COM_yaw_i input; phase input; y_avg output; acc_b input; Kp_vel input; vR input; vg_off input; y output
function [y_avg,y] = fcn(t,vel_COM_yaw_avg,vel_COM_yaw_i,phase,acc_b,Kp_vel,vR,vg_off)

Ts2 = 1/1000;
R = reshape(vR,[3,3]);

if t<5
    acc_b = zeros(3,1);
end

accel_wd = R * acc_b;
accel_wd = accel_wd + [0;0;-vg_off];


persistent vel_avg vel
if isempty(vel_avg)
    vel_avg = [0; 0; 0];
    vel = [0; 0; 0];
end

if t<5
    e_vel_avg = zeros(3,1);
else
    e_vel_avg = vel_avg - vel_COM_yaw_avg;
end

% phase
% 1/2/3/4 foot in contact
% otherwise four feet in contact
if phase == 0
    vel_COM_yaw = vel;
elseif phase == 1
    vel_COM_yaw = vel_COM_yaw_i(1:3);
elseif phase == 2
    vel_COM_yaw = vel_COM_yaw_i(4:6);
elseif phase == 3
    vel_COM_yaw = vel_COM_yaw_i(7:9);
elseif phase == 4
    vel_COM_yaw = vel_COM_yaw_i(10:12);
else
    vel_COM_yaw = vel_COM_yaw_avg;
end

if t<5
    e_dir = zeros(3,1);
else
    e_dir = vel - vel_COM_yaw;
end

qDot_avg = accel_wd - Kp_vel * e_vel_avg;
qDot = accel_wd - Kp_vel * e_dir;

vel_avg = vel_avg + qDot_avg * Ts2;
vel = vel + qDot * Ts2;

y_avg = vel_avg;
y = vel;

end

== matlab function ICRA_demo_ver2/Custom Detect Change ==
  data: u input; y output
function y = fcn(u)
%#codegen
persistent y_prev
if isempty(y_prev)
    y_prev = zeros(size(u));
end
y = zeros(size(u));

for ii=1:length(u)
    if u(ii)~=y_prev(ii)
        y(ii) = 1;
    end
end
y_prev = u;

== matlab function ICRA_demo_ver2/workspace Ctrl ==
  data: J_f_b output; p_f_b output; p_f_yaw output; p_h2f_yaw output; q_all input; dq_all input; vR_yaw input; pos_COM_yaw_avg output; v_h2f_b output; v_h2f_yaw output; vel_COM_yaw_avg output; wb input; vel_COM_yaw_i output; r_COM_yaw_i output
function [J_f_b,p_f_b,p_f_yaw,p_h2f_yaw,pos_COM_yaw_avg,v_h2f_b,v_h2f_yaw,...
          vel_COM_yaw_avg,vel_COM_yaw_i,r_COM_yaw_i] = ...
                workspacePDctrl(q_all, dq_all,vR_yaw,wb)

Ryaw = reshape(vR_yaw,[3,3]);

L = 0.3;    % body length
l1 = 0.14;   % link length
l2 = 0.17;
a = 0.045;   % torso width
b = 0.04;   % ABAD motor offset

% sign for four legs. sequence: FL,FR,HL,HR
sign_L = [1 1 -1 -1];
sign_ab = [1 -1 1 -1];

% initialize
p_hip_b = zeros(12,1);
p_f_b = zeros(12,1);
p_f_yaw = zeros(12,1);
p_h2f_b = zeros(12,1);
p_h2f_yaw = zeros(12,1);
J_f_b = zeros(36,1);
v_h2f_b = zeros(12,1);
v_h2f_yaw = zeros(12,1);

%%
for i_leg = 1:4
    params = [sign_L(i_leg)*L,l1,l2,sign_ab(i_leg)*[a b]];
    idx = 3*(i_leg-1) + (1:3);
    q_i_leg = q_all(idx);
    dq_i_leg = dq_all(idx);
    
    p_hip_b(idx) = [sign_L(i_leg)*L/2;sign_ab(i_leg)*a;0];
    p_f_b(idx) = fcn_p_(q_i_leg, params);
    p_f_yaw(idx) = Ryaw * p_f_b(idx);
    p_h2f_b(idx) = p_f_b(idx) - p_hip_b(idx);
    p_h2f_yaw(idx) = Ryaw * p_h2f_b(idx);
    
    J_f_b_temp = fcn_J_(q_i_leg, params);
    J_f_b((i_leg-1)*9+1:9*i_leg) = reshape(J_f_b_temp,[9,1]);
    
    v_h2f_b(idx) = J_f_b_temp * dq_i_leg;
    v_h2f_yaw(idx) = Ryaw * v_h2f_b(idx);
    
end


%% CoM position
pos_COM_b_1 = -p_f_b(1:3);
pos_COM_b_2 = -p_f_b(4:6);
pos_COM_b_3 = -p_f_b(7:9);
pos_COM_b_4 = -p_f_b(10:12);
pos_COM_b_avg = -1/4 * sum(reshape(p_f_b,[3,4]),2);
pos_COM_yaw_avg = Ryaw * pos_COM_b_avg;

% from foot to CoM
r_COM_yaw_1 = Ryaw * pos_COM_b_1;
r_COM_yaw_2 = Ryaw * pos_COM_b_2;
r_COM_yaw_3 = Ryaw * pos_COM_b_3;
r_COM_yaw_4 = Ryaw * pos_COM_b_4;
r_COM_yaw_i = [r_COM_yaw_1;r_COM_yaw_2;r_COM_yaw_3;r_COM_yaw_4];

%% CoM velocity in {W}
vel_COM_b_1 = - v_h2f_b(1:3);
vel_COM_b_2 = - v_h2f_b(4:6);
vel_COM_b_3 = - v_h2f_b(7:9);
vel_COM_b_4 = - v_h2f_b(10:12);
vel_COM_b = -1/4 * sum(reshape(v_h2f_b,[3,4]),2);

vel_COM_yaw_1 = Ryaw * Vec_to_Skew(wb) * pos_COM_b_1 + Ryaw * vel_COM_b_1;
vel_COM_yaw_2 = Ryaw * Vec_to_Skew(wb) * pos_COM_b_2 + Ryaw * vel_COM_b_2;
vel_COM_yaw_3 = Ryaw * Vec_to_Skew(wb) * pos_COM_b_3 + Ryaw * vel_COM_b_3;
vel_COM_yaw_4 = Ryaw * Vec_to_Skew(wb) * pos_COM_b_4 + Ryaw * vel_COM_b_4;
vel_COM_yaw_i = [vel_COM_yaw_1;vel_COM_yaw_2;vel_COM_yaw_3;vel_COM_yaw_4];
vel_COM_yaw_avg = Ryaw * Vec_to_Skew(wb) * pos_COM_b_avg + Ryaw * vel_COM_b;


end

function S = Vec_to_Skew(s)

S = zeros(3,3);
S(1,2) = -s(3);
S(1,3) = s(2);
S(2,1) = s(3);
S(2,3) = -s(1);
S(3,1) = -s(2);
S(3,2) = s(1);

end
